simulink model "Test_Arithmetic_Operation_Bit_Adder_Data_Out"  (R2023a)
settings: Solver=ode45  StartTime=0.0  StopTime=len  RelTol=1e-3  EnableMultiTasking=on
libraries: Arithmetic_Operations_Lib x1
settings Model: Creator=uzivatel  LastModifiedBy=Jozko Mrkvicka
settings SolverCC: AlgebraicLoopSolver=TrustRegion
settings DataIOCC: LimitDataPoints=on  SaveFormat=Array  ReturnWorkspaceOutputs=off
settings OptimizationCC: LifeSpan=inf
settings DebuggingCC: UnderspecifiedInitializationDetection=Classic  MergeDetectMultiDrivingBlocksExec=none  SolverPrmCheckMsg=warning  UnconnectedInputMsg=warning  UnconnectedOutputMsg=warning  UnconnectedLineMsg=warning  StateNameClashWarn=warning  SFUnexpectedBacktrackingDiag=warning  SFNoUnconditionalDefaultTransitionDiag=warning  ArithmeticOperatorsInVariantConditions=warning
settings HardwareCC: ProdBitPerPointer=32  ProdBitPerSizeT=32  ProdBitPerPtrDiffT=32  ProdLargestAtomicFloat=None  ProdIntDivRoundTo=Undefined  ProdEndianess=Unspecified  ProdWordSize=32  ProdHWDeviceType=32-bit Generic
settings ModelReferenceCC: EnableRefExpFcnMdlSchedulingChecks=on  PropagateSignalLabelsOutOfModel=off
settings SFSimCC: SimUseLocalCustomCode=off  CustomCodeUndefinedFunction=UseInterfaceOnly
settings RTWCC: RTWUseLocalCustomCode=off
settings CodeAppCC: StateflowObjectComments=on
settings GRTTargetCC: TargetLangStandard=C89/C90 (ANSI)
settings ConfigComp: CovMetricSettings=dw  CovSaveCumulativeToWorkspaceVar=on  CovSaveSingleToWorkspaceVar=on  CovExternalEMLEnable=off

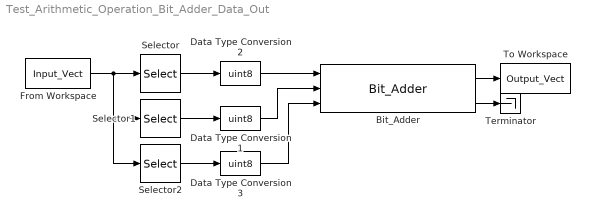
== system Test_Arithmetic_Operation_Bit_Adder_Data_Out ==
  Bit_Adder : Arithmetic_Operations_Lib/Bit_Adder  SystemSampleTime=-1  VariantActivationTime=update diagram  Latency=0  AutoFrameSizeCalculation=off
  Data Type Conversion1 : DataTypeConversion  OutDataTypeStr=uint8  SaturateOnIntegerOverflow=off  RndMeth=Floor
  Data Type Conversion2 : DataTypeConversion  OutDataTypeStr=uint8  SaturateOnIntegerOverflow=off  RndMeth=Floor
  Data Type Conversion3 : DataTypeConversion  OutDataTypeStr=uint8  SaturateOnIntegerOverflow=off  RndMeth=Floor
  From Workspace : FromWorkspace  VariableName=Input_Vect  SampleTime=1  Interpolate=off  ZeroCross=off  OutputAfterFinalValue=Holding final value
  Selector : Selector  IndexMode=Zero-based  InputPortWidth=3  SampleTime=1  IndexOptions=Index vector (dialog)  Indices=0  OutputSizes=1
  Selector1 : Selector  IndexMode=Zero-based  InputPortWidth=3  SampleTime=1  IndexOptions=Index vector (dialog)  Indices=1  OutputSizes=1
  Selector2 : Selector  IndexMode=Zero-based  InputPortWidth=3  SampleTime=1  IndexOptions=Index vector (dialog)  Indices=2  OutputSizes=1
  Terminator : Terminator
  To Workspace : ToWorkspace  VariableName=Output_Vect  SampleTime=1
  wires:
  From Workspace/1 -> Selector2/1, Selector1/1, Selector/1
  Selector1/1 -> Data Type Conversion1/1
  Selector/1 -> Data Type Conversion2/1
  Data Type Conversion2/1 -> Bit_Adder/1
  Bit_Adder/2 -> Terminator/1
  Bit_Adder/1 -> To Workspace/1
  Selector2/1 -> Data Type Conversion3/1
  Data Type Conversion1/1 -> Bit_Adder/2
  Data Type Conversion3/1 -> Bit_Adder/3
